simulink model "CRDI_Integrated_Model0707"  (R2019a)
settings: configuration reference "cs1" (kept outside this file)
PreLoadFcn:
  | Configaration_Setting
undefined symbols (not defined in the file or in its folder): AreaOfOrifice_Constant, CcConstant_0, CcConstant_1, Constant_0, Constant_1, Constant_One, Divide_by_100, Error_code_101, Error_code_102, FilterConstant_0, FilterConstant_1, FilterConstant_100, FilterConstant_5, FilterConstant_50, Final_Crank_Angle, Fuel_Discharge, HPPConstant1, HPPConstant2, LPPConstant_0, LPPConstant_1, LPPConstant_10, LPPConstant_3, Main_TgrAng_Inj1, Main_TgrAng_Inj2, Main_TgrAng_Inj3, Main_TgrAng_Inj4, MeterToLiter_Conversion, Orifice_Diameter, Percentage, Pi_value, Post_TgrAng_Inj1, Post_TgrAng_Inj2, Post_TgrAng_Inj3, Post_TgrAng_Inj4, Pre_TgrAng_Inj1, Pre_TgrAng_Inj2, Pre_TgrAng_Inj3, Pre_TgrAng_Inj4, Re_Rounding_Constant, Required_PulseConstant1, Required_PulseConstant2, Required_PulseConstant3, Required_PulseConstant4, resistance_constant, Rounding_Constant_100, Scalling_Factor, Unit_Angle_Compare, Velocity_MulFactor1, Velocity_MulFactor2, Velocity_MulFactor3, Zero_Pulse
libraries: simulink x4
(part 2 of 2)

== system CRDI_Integrated_Model0707/CRDI/Injector_Model/injector1/mainInj1 ==
  Angle : Inport  OutDataTypeStr=single
  Total_On_Time_of_Injector : Inport  Port=2  OutDataTypeStr=single
  Time_For_1_Degree : Inport  Port=3  OutDataTypeStr=single
  Add : Sum  AccumDataTypeStr=single
      settings: AttributesFormatString=AccumDataTypeStr=%<AccumDataTypeStr>
  Constant : Constant  Value=Constant_0
  Constant1 : Constant  Value=Constant_1
  Constant4 : Constant  Value=Main_TgrAng_Inj1
  Constant6 : Constant  Value=Constant_0
  Divide : Product  Inputs=*/  OutDataTypeStr=single
  Logical Operator : Logic  Inputs=3  AllPortsSameDT=off  OutDataTypeStr=boolean
  Relational Operator : RelationalOperator  OutDataTypeStr=boolean  RndMeth=Simplest
  Relational Operator1 : RelationalOperator  Operator=<=  OutDataTypeStr=boolean  RndMeth=Simplest
  Relational Operator2 : RelationalOperator  Operator=>  OutDataTypeStr=boolean  RndMeth=Simplest
  Relational Operator3 : RelationalOperator  Operator=>  OutDataTypeStr=boolean  RndMeth=Simplest
  Switch : Switch  Criteria=u2 ~= 0
  OnPulse_Main : Outport
  wires:
  Switch/1 -> Divide/2  "Time_Of_1_Degree"
  Constant1/1 -> Switch/3  "constant"
  Time_For_1_Degree/1 -> Switch/1, Relational Operator3/1
  [onTinj1] -> Relational Operator2/1
  Total_On_Time_of_Injector/1 -> [onTinj1], Divide/1
  Constant4/1 -> [TrigerAngle], Add/1  "TrigerAngle"
  [TrigerAngle] -> Relational Operator/2
  Relational Operator2/1 -> Logical Operator/3  "Speed_Zero_Or_Not"
  Constant/1 -> Relational Operator2/2  "constant"
  Logical Operator/1 -> OnPulse_Main/1  "OnPulse_Main"
  Divide/1 -> Add/2  "Time_For_On_Pulse"
  Angle/1 -> Relational Operator/1, Relational Operator1/1
  Add/1 -> Relational Operator1/2  "Total_On_Degree"
  Relational Operator/1 -> Logical Operator/1  "Firing_Angle_start"
  Relational Operator1/1 -> Logical Operator/2  "Firing_Angle_Off"
  Relational Operator3/1 -> Switch/2  "Non_Zero_Num"
  Constant6/1 -> Relational Operator3/2  "constant"

== system CRDI_Integrated_Model0707/CRDI/Injector_Model/injector1/postInj1 ==
  Angle : Inport  OutDataTypeStr=single
  Total_On_Time_of_Injector : Inport  Port=2  OutDataTypeStr=single
  Time_for_1_Degree : Inport  Port=3  OutDataTypeStr=single
  Add : Sum  AccumDataTypeStr=single
      settings: AttributesFormatString=AccumDataTypeStr=%<AccumDataTypeStr>
  Constant : Constant  Value=Constant_0
  Constant1 : Constant  Value=Constant_1
  Constant5 : Constant  Value=Post_TgrAng_Inj1
  Constant6 : Constant  Value=Constant_0
  Divide : Product  Inputs=*/  OutDataTypeStr=single
  Logical Operator : Logic  Inputs=3  AllPortsSameDT=off  OutDataTypeStr=boolean
  Relational Operator : RelationalOperator  OutDataTypeStr=boolean  RndMeth=Simplest
  Relational Operator1 : RelationalOperator  Operator=<=  OutDataTypeStr=boolean  RndMeth=Simplest
  Relational Operator2 : RelationalOperator  Operator=>  OutDataTypeStr=boolean  RndMeth=Simplest
  Relational Operator3 : RelationalOperator  Operator=>  OutDataTypeStr=boolean  RndMeth=Simplest
  Switch : Switch  Criteria=u2 ~= 0
  OnPulse_Post : Outport
  wires:
  Time_for_1_Degree/1 -> Relational Operator3/1, Switch/1
  Constant1/1 -> Switch/3  "constant"
  Switch/1 -> Divide/2  "Time_Of_1_Degree"
  Constant5/1 -> Add/1, [TrigerAngle]  "TrigerAngle"
  [TrigerAngle] -> Relational Operator/2
  [onTinj1] -> Relational Operator2/1
  Total_On_Time_of_Injector/1 -> [onTinj1], Divide/1
  Relational Operator2/1 -> Logical Operator/3  "Speed_Zero_Or_Not"
  Constant/1 -> Relational Operator2/2  "constant"
  Logical Operator/1 -> OnPulse_Post/1  "OnPulse_Post"
  Relational Operator1/1 -> Logical Operator/2  "Firing_Angle_Off"
  Relational Operator/1 -> Logical Operator/1  "Firing_Angle_start"
  Add/1 -> Relational Operator1/2  "Total_On_Degree"
  Angle/1 -> Relational Operator/1, Relational Operator1/1
  Divide/1 -> Add/2  "Time_For_On_Pulse"
  Relational Operator3/1 -> Switch/2  "Non_Zero_Num"
  Constant6/1 -> Relational Operator3/2  "constant"

== system CRDI_Integrated_Model0707/CRDI/Injector_Model/injector2/PreInj1 ==
  Angle : Inport  OutDataTypeStr=single
  Total_On_Time_of_Injector : Inport  Port=2  OutDataTypeStr=single
  Time_For_1_Degree : Inport  Port=3  OutDataTypeStr=single
  Add : Sum  AccumDataTypeStr=single
      settings: AttributesFormatString=AccumDataTypeStr=%<AccumDataTypeStr>
  Constant : Constant  Value=Constant_0
  Constant1 : Constant  Value=Constant_1
  Constant2 : Constant  Value=Pre_TgrAng_Inj3  OutDataTypeStr=single
  Constant6 : Constant  Value=Constant_0
  Divide : Product  Inputs=*/  OutDataTypeStr=single
  Logical Operator : Logic  Inputs=3  AllPortsSameDT=off  OutDataTypeStr=boolean
  Relational Operator : RelationalOperator  OutDataTypeStr=boolean  RndMeth=Simplest
  Relational Operator1 : RelationalOperator  Operator=<=  OutDataTypeStr=boolean  RndMeth=Simplest
  Relational Operator2 : RelationalOperator  Operator=>  OutDataTypeStr=boolean  RndMeth=Simplest
  Relational Operator3 : RelationalOperator  Operator=>  OutDataTypeStr=boolean  RndMeth=Simplest
  Switch : Switch  Criteria=u2 ~= 0
  OnPulse_Pre : Outport
  wires:
  Constant1/1 -> Switch/3  "constant"
  Switch/1 -> Divide/2  "Time_Of_1_Degree"
  Constant2/1 -> [TrigerAngle], Add/1  "TrigerAngle"
  [TrigerAngle] -> Relational Operator/2
  [onTinj] -> Relational Operator2/1
  Total_On_Time_of_Injector/1 -> [onTinj], Divide/1
  Constant/1 -> Relational Operator2/2  "constant"
  Relational Operator2/1 -> Logical Operator/3  "Speed_Zero_Or_Not"
  Logical Operator/1 -> OnPulse_Pre/1  "OnPulse_Pre"
  Relational Operator1/1 -> Logical Operator/2  "Firing_Angle_Off"
  Relational Operator/1 -> Logical Operator/1  "Firing_Angle_start"
  Add/1 -> Relational Operator1/2  "Total_On_Degree"
  Angle/1 -> Relational Operator1/1, Relational Operator/1
  Divide/1 -> Add/2  "Time_For_On_Pulse"
  Relational Operator3/1 -> Switch/2  "Non_Zero_Num"
  Constant6/1 -> Relational Operator3/2  "constant"
  Time_For_1_Degree/1 -> Switch/1, Relational Operator3/1

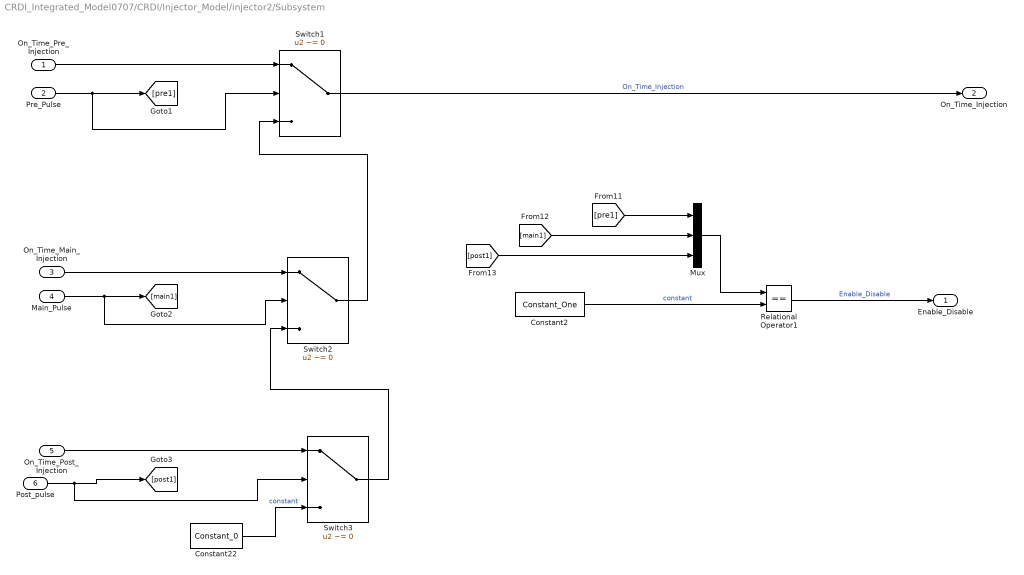
== system CRDI_Integrated_Model0707/CRDI/Injector_Model/injector2/Subsystem ==
  On_Time_Pre_Injection : Inport
  Pre_Pulse : Inport  Port=2
  On_Time_Main_Injection : Inport  Port=3
  Main_Pulse : Inport  Port=4
  On_Time_Post_Injection : Inport  Port=5
  Post_pulse : Inport  Port=6
  Constant2 : Constant  Value=Constant_One  OutDataTypeStr=single
  Constant22 : Constant  Value=Constant_0  OutDataTypeStr=single
  Mux : Mux  Inputs=3
  Relational Operator1 : RelationalOperator  Operator===  OutDataTypeStr=boolean  RndMeth=Simplest
  Switch1 : Switch  Criteria=u2 ~= 0
  Switch2 : Switch  Criteria=u2 ~= 0
  Switch3 : Switch  Criteria=u2 ~= 0
  Enable_Disable : Outport
  On_Time_Injection : Outport  Port=2
  wires:
  Post_pulse/1 -> [post1], Switch3/2
  On_Time_Post_Injection/1 -> Switch3/1
  Main_Pulse/1 -> [main1], Switch2/2
  On_Time_Main_Injection/1 -> Switch2/1
  Pre_Pulse/1 -> [pre1], Switch1/2
  On_Time_Pre_Injection/1 -> Switch1/1
  Switch1/1 -> On_Time_Injection/1  "On_Time_Injection"
  Relational Operator1/1 -> Enable_Disable/1  "Enable_Disable"
  Constant22/1 -> Switch3/3  "constant"
  [main1] -> Mux/2
  Switch3/1 -> Switch2/3
  Switch2/1 -> Switch1/3
  Mux/1 -> Relational Operator1/1
  [pre1] -> Mux/1
  [post1] -> Mux/3
  Constant2/1 -> Relational Operator1/2  "constant"

== system CRDI_Integrated_Model0707/CRDI/Injector_Model/injector2/Subsystem7 ==
  On_Time : Inport
  Enable : EnablePort  StatesWhenEnabling=reset  PropagateVarSize=During execution
  Add : Sum  AccumDataTypeStr=single
      settings: AttributesFormatString=AccumDataTypeStr=%<AccumDataTypeStr>
  Constant : Constant  Value=Re_Rounding_Constant  OutDataTypeStr=single
  Relational Operator : RelationalOperator  Operator=<=  OutDataTypeStr=boolean  RndMeth=Simplest
  Subsystem : Subsystem  Commented=on
  Unit Delay : UnitDelay  SampleTime=-1  HasFrameUpgradeWarning=on
  Final_Inj_Pulse : Outport  OutDataTypeStr=boolean
  wires:
  Relational Operator/1 -> Final_Inj_Pulse/1  "Final_Inj_Pulse"
  Unit Delay/1 -> Add/1
  Constant/1 -> Add/2  "constant"
  Add/1 -> Relational Operator/1, Unit Delay/1
  On_Time/1 -> Relational Operator/2

== system CRDI_Integrated_Model0707/CRDI/Injector_Model/injector2/mainInj1 ==
  Angle : Inport  OutDataTypeStr=single
  Total_On_Time_of_Injector : Inport  Port=2  OutDataTypeStr=single
  Time_For_1_Degree : Inport  Port=3  OutDataTypeStr=single
  Add : Sum  AccumDataTypeStr=single
      settings: AttributesFormatString=AccumDataTypeStr=%<AccumDataTypeStr>
  Constant : Constant  Value=Constant_0
  Constant1 : Constant  Value=Constant_1
  Constant4 : Constant  Value=Main_TgrAng_Inj3
  Constant6 : Constant  Value=Constant_0
  Divide : Product  Inputs=*/  OutDataTypeStr=single
  Logical Operator : Logic  Inputs=3  AllPortsSameDT=off  OutDataTypeStr=boolean
  Relational Operator : RelationalOperator  OutDataTypeStr=boolean  RndMeth=Simplest
  Relational Operator1 : RelationalOperator  Operator=<=  OutDataTypeStr=boolean  RndMeth=Simplest
  Relational Operator2 : RelationalOperator  Operator=>  OutDataTypeStr=boolean  RndMeth=Simplest
  Relational Operator3 : RelationalOperator  Operator=>  OutDataTypeStr=boolean  RndMeth=Simplest
  Switch : Switch  Criteria=u2 ~= 0
  OnPulse_Main : Outport
  wires:
  Switch/1 -> Divide/2  "Time_Of_1_Degree"
  Constant1/1 -> Switch/3  "constant"
  [onTinj1] -> Relational Operator2/1
  Total_On_Time_of_Injector/1 -> [onTinj1], Divide/1
  Constant4/1 -> [TrigerAngle], Add/1  "TrigerAngle"
  [TrigerAngle] -> Relational Operator/2
  Relational Operator2/1 -> Logical Operator/3  "Speed_Zero_Or_Not"
  Constant/1 -> Relational Operator2/2  "constant"
  Logical Operator/1 -> OnPulse_Main/1  "OnPulse_Main"
  Divide/1 -> Add/2  "Time_For_On_Pulse"
  Angle/1 -> Relational Operator/1, Relational Operator1/1
  Add/1 -> Relational Operator1/2  "Total_On_Degree"
  Relational Operator/1 -> Logical Operator/1  "Firing_Angle_start"
  Relational Operator1/1 -> Logical Operator/2  "Firing_Angle_Off"
  Relational Operator3/1 -> Switch/2  "Non_Zero_Num"
  Constant6/1 -> Relational Operator3/2  "constant"
  Time_For_1_Degree/1 -> Switch/1, Relational Operator3/1

== system CRDI_Integrated_Model0707/CRDI/Injector_Model/injector2/postInj1 ==
  Angle : Inport  OutDataTypeStr=single
  Total_On_Time_of_Injector : Inport  Port=2  OutDataTypeStr=single
  Time_for_1_Degree : Inport  Port=3  OutDataTypeStr=single
  Add : Sum  AccumDataTypeStr=single
      settings: AttributesFormatString=AccumDataTypeStr=%<AccumDataTypeStr>
  Constant : Constant  Value=Constant_0
  Constant1 : Constant  Value=Constant_1
  Constant5 : Constant  Value=Post_TgrAng_Inj3
  Constant6 : Constant  Value=Constant_0
  Divide : Product  Inputs=*/  OutDataTypeStr=single
  Logical Operator : Logic  Inputs=3  AllPortsSameDT=off  OutDataTypeStr=boolean
  Relational Operator : RelationalOperator  OutDataTypeStr=boolean  RndMeth=Simplest
  Relational Operator1 : RelationalOperator  Operator=<=  OutDataTypeStr=boolean  RndMeth=Simplest
  Relational Operator2 : RelationalOperator  Operator=>  OutDataTypeStr=boolean  RndMeth=Simplest
  Relational Operator3 : RelationalOperator  Operator=>  OutDataTypeStr=boolean  RndMeth=Simplest
  Switch : Switch  Criteria=u2 ~= 0
  OnPulse_Post : Outport
  wires:
  Constant1/1 -> Switch/3  "constant"
  Switch/1 -> Divide/2  "Time_Of_1_Degree"
  Constant5/1 -> Add/1, [TrigerAngle]  "TrigerAngle"
  [TrigerAngle] -> Relational Operator/2
  [onTinj1] -> Relational Operator2/1
  Total_On_Time_of_Injector/1 -> [onTinj1], Divide/1
  Relational Operator2/1 -> Logical Operator/3  "Speed_Zero_Or_Not"
  Constant/1 -> Relational Operator2/2  "constant"
  Logical Operator/1 -> OnPulse_Post/1  "OnPulse_Post"
  Relational Operator1/1 -> Logical Operator/2  "Firing_Angle_Off"
  Relational Operator/1 -> Logical Operator/1  "Firing_Angle_start"
  Add/1 -> Relational Operator1/2  "Total_On_Degree"
  Angle/1 -> Relational Operator/1, Relational Operator1/1
  Divide/1 -> Add/2  "Time_For_On_Pulse"
  Relational Operator3/1 -> Switch/2  "Non_Zero_Num"
  Constant6/1 -> Relational Operator3/2  "constant"
  Time_for_1_Degree/1 -> Switch/1, Relational Operator3/1

== system CRDI_Integrated_Model0707/CRDI/Injector_Model/injector3/PreInj1 ==
  Angle : Inport  OutDataTypeStr=single
  Total_On_Time_of_Injector : Inport  Port=2  OutDataTypeStr=single
  Time_For_1_Degree : Inport  Port=3  OutDataTypeStr=single
  Add : Sum  AccumDataTypeStr=single
      settings: AttributesFormatString=AccumDataTypeStr=%<AccumDataTypeStr>
  Constant : Constant  Value=Constant_0
  Constant1 : Constant  Value=Constant_1
  Constant6 : Constant  Value=Constant_0
  Constant9 : Constant  Value=Pre_TgrAng_Inj2  OutDataTypeStr=single
  Divide : Product  Inputs=*/  OutDataTypeStr=single
  Logical Operator : Logic  Inputs=3  AllPortsSameDT=off  OutDataTypeStr=boolean
  Relational Operator : RelationalOperator  OutDataTypeStr=boolean  RndMeth=Simplest
  Relational Operator1 : RelationalOperator  Operator=<=  OutDataTypeStr=boolean  RndMeth=Simplest
  Relational Operator2 : RelationalOperator  Operator=>  OutDataTypeStr=boolean  RndMeth=Simplest
  Relational Operator3 : RelationalOperator  Operator=>  OutDataTypeStr=boolean  RndMeth=Simplest
  Switch : Switch  Criteria=u2 ~= 0
  OnPulse_Pre : Outport
  wires:
  Time_For_1_Degree/1 -> Switch/1, Relational Operator3/1
  Constant1/1 -> Switch/3  "constant"
  Switch/1 -> Divide/2  "Time_Of_1_Degree"
  Constant9/1 -> [TrigerAngle], Add/1  "TrigerAngle"
  [TrigerAngle] -> Relational Operator/2
  [onTinj] -> Relational Operator2/1
  Total_On_Time_of_Injector/1 -> [onTinj], Divide/1
  Constant/1 -> Relational Operator2/2  "constant"
  Relational Operator2/1 -> Logical Operator/3  "Speed_Zero_Or_Not"
  Logical Operator/1 -> OnPulse_Pre/1  "OnPulse_Pre"
  Relational Operator1/1 -> Logical Operator/2  "Firing_Angle_Off"
  Relational Operator/1 -> Logical Operator/1  "Firing_Angle_start"
  Add/1 -> Relational Operator1/2  "Total_On_Degree"
  Angle/1 -> Relational Operator1/1, Relational Operator/1
  Divide/1 -> Add/2  "Time_For_On_Pulse"
  Relational Operator3/1 -> Switch/2  "Non_Zero_Num"
  Constant6/1 -> Relational Operator3/2  "constant"

== system CRDI_Integrated_Model0707/CRDI/Injector_Model/injector3/Subsystem ==
  On_Time_Pre_Injection : Inport
  Pre_Pulse : Inport  Port=2
  On_Time_Main_Injection : Inport  Port=3
  Main_Pulse : Inport  Port=4
  On_Time_Post_Injection : Inport  Port=5
  Post_pulse : Inport  Port=6
  Constant2 : Constant  Value=Constant_One  OutDataTypeStr=single
  Constant22 : Constant  Value=Constant_0  OutDataTypeStr=single
  Mux : Mux  Inputs=3
  Relational Operator1 : RelationalOperator  Operator===  OutDataTypeStr=boolean  RndMeth=Simplest
  Switch1 : Switch  Criteria=u2 ~= 0
  Switch2 : Switch  Criteria=u2 ~= 0
  Switch3 : Switch  Criteria=u2 ~= 0
  Enable_Disable : Outport
  On_Time_Injection : Outport  Port=2
  wires:
  Post_pulse/1 -> [post1], Switch3/2
  On_Time_Post_Injection/1 -> Switch3/1
  Main_Pulse/1 -> [main1], Switch2/2
  On_Time_Main_Injection/1 -> Switch2/1
  Pre_Pulse/1 -> [pre1], Switch1/2
  On_Time_Pre_Injection/1 -> Switch1/1
  Switch1/1 -> On_Time_Injection/1  "On_Time_Injection"
  Relational Operator1/1 -> Enable_Disable/1  "Enable_Disable"
  Constant22/1 -> Switch3/3  "constant"
  [main1] -> Mux/2
  Constant2/1 -> Relational Operator1/2  "constant"
  Switch3/1 -> Switch2/3
  Switch2/1 -> Switch1/3
  Mux/1 -> Relational Operator1/1
  [pre1] -> Mux/1
  [post1] -> Mux/3

== system CRDI_Integrated_Model0707/CRDI/Injector_Model/injector3/Subsystem7 ==
  On_Time : Inport
  Enable : EnablePort  StatesWhenEnabling=reset  PropagateVarSize=During execution
  Add : Sum  AccumDataTypeStr=single
      settings: AttributesFormatString=AccumDataTypeStr=%<AccumDataTypeStr>
  Constant : Constant  Value=Re_Rounding_Constant  OutDataTypeStr=single
  Relational Operator : RelationalOperator  Operator=<=  OutDataTypeStr=boolean  RndMeth=Simplest
  Subsystem : Subsystem  Commented=on
  Unit Delay : UnitDelay  SampleTime=-1  HasFrameUpgradeWarning=on
  Final_Inj_Pulse : Outport  OutDataTypeStr=boolean
  wires:
  Relational Operator/1 -> Final_Inj_Pulse/1  "Final_Inj_Pulse"
  Unit Delay/1 -> Add/1
  Constant/1 -> Add/2  "constant"
  Add/1 -> Relational Operator/1, Unit Delay/1
  On_Time/1 -> Relational Operator/2

== system CRDI_Integrated_Model0707/CRDI/Injector_Model/injector3/mainInj1 ==
  Angle : Inport  OutDataTypeStr=single
  Total_On_Time_of_Injector : Inport  Port=2  OutDataTypeStr=single
  Time_For_1_Degree : Inport  Port=3  OutDataTypeStr=single
  Add : Sum  AccumDataTypeStr=single
      settings: AttributesFormatString=AccumDataTypeStr=%<AccumDataTypeStr>
  Constant : Constant  Value=Constant_0
  Constant1 : Constant  Value=Constant_1
  Constant11 : Constant  Value=Main_TgrAng_Inj2  OutDataTypeStr=single
  Constant6 : Constant  Value=Constant_0
  Divide : Product  Inputs=*/  OutDataTypeStr=single
  Logical Operator : Logic  Inputs=3  AllPortsSameDT=off  OutDataTypeStr=boolean
  Relational Operator : RelationalOperator  OutDataTypeStr=boolean  RndMeth=Simplest
  Relational Operator1 : RelationalOperator  Operator=<=  OutDataTypeStr=boolean  RndMeth=Simplest
  Relational Operator2 : RelationalOperator  Operator=>  OutDataTypeStr=boolean  RndMeth=Simplest
  Relational Operator3 : RelationalOperator  Operator=>  OutDataTypeStr=boolean  RndMeth=Simplest
  Switch : Switch  Criteria=u2 ~= 0
  OnPulse_Main : Outport
  wires:
  Switch/1 -> Divide/2  "Time_Of_1_Degree"
  Constant1/1 -> Switch/3  "constant"
  Time_For_1_Degree/1 -> Relational Operator3/1, Switch/1
  [onTinj1] -> Relational Operator2/1
  Total_On_Time_of_Injector/1 -> [onTinj1], Divide/1
  Constant11/1 -> [TrigerAngle], Add/1  "TrigerAngle"
  [TrigerAngle] -> Relational Operator/2
  Relational Operator2/1 -> Logical Operator/3  "Speed_Zero_Or_Not"
  Constant/1 -> Relational Operator2/2  "constant"
  Logical Operator/1 -> OnPulse_Main/1  "OnPulse_Main"
  Divide/1 -> Add/2  "Time_For_On_Pulse"
  Angle/1 -> Relational Operator/1, Relational Operator1/1
  Add/1 -> Relational Operator1/2  "Total_On_Degree"
  Relational Operator/1 -> Logical Operator/1  "Firing_Angle_start"
  Relational Operator1/1 -> Logical Operator/2  "Firing_Angle_Off"
  Relational Operator3/1 -> Switch/2  "Non_Zero_Num"
  Constant6/1 -> Relational Operator3/2  "constant"

== system CRDI_Integrated_Model0707/CRDI/Injector_Model/injector3/postInj1 ==
  Angle : Inport  OutDataTypeStr=single
  Total_On_Time_of_Injector : Inport  Port=2  OutDataTypeStr=single
  Time_for_1_Degree : Inport  Port=3  OutDataTypeStr=single
  Add : Sum  AccumDataTypeStr=single
      settings: AttributesFormatString=AccumDataTypeStr=%<AccumDataTypeStr>
  Constant : Constant  Value=Constant_0
  Constant1 : Constant  Value=Constant_1
  Constant12 : Constant  Value=Post_TgrAng_Inj2
  Constant6 : Constant  Value=Constant_0
  Divide : Product  Inputs=*/  OutDataTypeStr=single
  Logical Operator : Logic  Inputs=3  AllPortsSameDT=off  OutDataTypeStr=boolean
  Relational Operator : RelationalOperator  OutDataTypeStr=boolean  RndMeth=Simplest
  Relational Operator1 : RelationalOperator  Operator=<=  OutDataTypeStr=boolean  RndMeth=Simplest
  Relational Operator2 : RelationalOperator  Operator=>  OutDataTypeStr=boolean  RndMeth=Simplest
  Relational Operator3 : RelationalOperator  Operator=>  OutDataTypeStr=boolean  RndMeth=Simplest
  Switch : Switch  Criteria=u2 ~= 0
  OnPulse_Post : Outport
  wires:
  Time_for_1_Degree/1 -> Relational Operator3/1, Switch/1
  Constant1/1 -> Switch/3  "constant"
  Switch/1 -> Divide/2  "Time_Of_1_Degree"
  Constant12/1 -> Add/1, [TrigerAngle]  "TrigerAngle"
  [TrigerAngle] -> Relational Operator/2
  [onTinj1] -> Relational Operator2/1
  Total_On_Time_of_Injector/1 -> [onTinj1], Divide/1
  Relational Operator2/1 -> Logical Operator/3  "Speed_Zero_Or_Not"
  Constant/1 -> Relational Operator2/2  "constant"
  Logical Operator/1 -> OnPulse_Post/1  "OnPulse_Post"
  Relational Operator1/1 -> Logical Operator/2  "Firing_Angle_Off"
  Relational Operator/1 -> Logical Operator/1  "Firing_Angle_start"
  Add/1 -> Relational Operator1/2  "Total_On_Degree"
  Angle/1 -> Relational Operator/1, Relational Operator1/1
  Divide/1 -> Add/2  "Time_For_On_Pulse"
  Relational Operator3/1 -> Switch/2  "Non_Zero_Num"
  Constant6/1 -> Relational Operator3/2  "constant"

== system CRDI_Integrated_Model0707/CRDI/Injector_Model/injector4/MainInj4 ==
  angle : Inport  OutDataTypeStr=single
  total_on_time_of_injector : Inport  Port=2  OutDataTypeStr=single
  time_for_1_degree : Inport  Port=3  OutDataTypeStr=single
  speed : Inport  Port=4  OutDataTypeStr=single
  Add : Sum  AccumDataTypeStr=single
      settings: AttributesFormatString=AccumDataTypeStr=%<AccumDataTypeStr>
  Constant : Constant  OutDataTypeStr=single
  Constant1 : Constant  Value=Constant_0
  Constant2 : Constant  Value=Constant_1
  Constant23 : Constant  Value=Main_TgrAng_Inj4
  Constant6 : Constant  Value=Constant_0
  Display : Display
  Display1 : Display
  Display2 : Display
  Divide : Product  Inputs=*/  OutDataTypeStr=single
  Relational Operator : RelationalOperator  Operator===  OutDataTypeStr=boolean  RndMeth=Simplest
  Relational Operator1 : RelationalOperator  Operator=<=  OutDataTypeStr=boolean  RndMeth=Simplest
  Relational Operator2 : RelationalOperator  Operator=>  OutDataTypeStr=boolean  RndMeth=Simplest
  Relational Operator3 : RelationalOperator  Operator=>  OutDataTypeStr=boolean  RndMeth=Simplest
  Switch : Switch  Criteria=u2 ~= 0
  OnPulse_Post : Outport  OutDataTypeStr=boolean
  wires:
  total_on_time_of_injector/1 -> Divide/1
  Divide/1 -> Add/2  "Time_For_On_Pulse"
  angle/1 -> Relational Operator1/1, Relational Operator/1
  Constant23/1 -> Relational Operator/2  "TrigerAngle"
  Add/1 -> Relational Operator1/2  "Total_On_Degree"
  Constant/1 -> Add/1  "constant"
  Constant1/1 -> Relational Operator2/2  "constant"
  speed/1 -> Relational Operator2/1
  Relational Operator/1 -> Display/1  "Equal"
  Relational Operator2/1 -> Display2/1  "Speed_Zero"
  Relational Operator1/1 -> OnPulse_Post/1, Display1/1  "OnPulse_Post"
  Switch/1 -> Divide/2
  Constant2/1 -> Switch/3  "constant"
  time_for_1_degree/1 -> Relational Operator3/1, Switch/1
  Relational Operator3/1 -> Switch/2  "Non_Zero_Num"
  Constant6/1 -> Relational Operator3/2  "constant"

== system CRDI_Integrated_Model0707/CRDI/Injector_Model/injector4/On_Time_Injector ==
  On_Time_Pre_Inj : Inport
  Pre_Pulse : Inport  Port=2
  On_Time_Main_Inj : Inport  Port=3
  Main_Pulse : Inport  Port=4
  On_Time_Post_Inj : Inport  Port=5
  Post_pulse : Inport  Port=6
  Constant22 : Constant  Value=Constant_0  OutDataTypeStr=single
  Constant3 : Constant  Value=Constant_One  OutDataTypeStr=single
  Mux : Mux  Inputs=3
  Relational Operator1 : RelationalOperator  Operator===  OutDataTypeStr=boolean  RndMeth=Simplest
  Switch1 : Switch  Criteria=u2 ~= 0
  Switch2 : Switch  Criteria=u2 ~= 0
  Switch3 : Switch  Criteria=u2 ~= 0
  Enable_Disable : Outport
  On_Time_injector : Outport  Port=2
  wires:
  [pre1] -> Mux/1
  [main1] -> Mux/2
  Switch3/1 -> Switch2/3  "OTPI"
  Post_pulse/1 -> Switch3/2, [post1]
  Switch1/1 -> On_Time_injector/1  "On_Time_injector"
  [post1] -> Mux/3
  Relational Operator1/1 -> Enable_Disable/1  "Enable_Disable"
  Main_Pulse/1 -> Switch2/2, [main1]
  On_Time_Pre_Inj/1 -> Switch1/1
  Pre_Pulse/1 -> Switch1/2, [pre1]
  Constant22/1 -> Switch3/3  "constant"
  Constant3/1 -> Relational Operator1/2  "constant"
  Switch2/1 -> Switch1/3  "OTMI"
  Mux/1 -> Relational Operator1/1  "Bus"
  On_Time_Main_Inj/1 -> Switch2/1
  On_Time_Post_Inj/1 -> Switch3/1

== system CRDI_Integrated_Model0707/CRDI/Injector_Model/injector4/PostInj4 ==
  angle : Inport  OutDataTypeStr=single
  total_on_time_of_injector : Inport  Port=2  OutDataTypeStr=single
  time_for_1_degree : Inport  Port=3  OutDataTypeStr=single
  Add : Sum  AccumDataTypeStr=single
      settings: AttributesFormatString=AccumDataTypeStr=%<AccumDataTypeStr>
  Constant : Constant  Value=Constant_0
  Constant1 : Constant  Value=Constant_1
  Constant24 : Constant  Value=Post_TgrAng_Inj4
  Constant6 : Constant  Value=Constant_0
  Divide : Product  Inputs=*/  OutDataTypeStr=single
  Logical Operator : Logic  Inputs=3  AllPortsSameDT=off  OutDataTypeStr=boolean
  Relational Operator : RelationalOperator  OutDataTypeStr=boolean  RndMeth=Simplest
  Relational Operator1 : RelationalOperator  Operator=<=  OutDataTypeStr=boolean  RndMeth=Simplest
  Relational Operator2 : RelationalOperator  Operator=>  OutDataTypeStr=boolean  RndMeth=Simplest
  Relational Operator3 : RelationalOperator  Operator=>  OutDataTypeStr=boolean  RndMeth=Simplest
  Switch : Switch  Criteria=u2 ~= 0
  OnPulse_Post : Outport  OutDataTypeStr=boolean
  wires:
  Logical Operator/1 -> OnPulse_Post/1  "OnPulse_Post"
  Relational Operator1/1 -> Logical Operator/2  "Rel_Op"
  Relational Operator/1 -> Logical Operator/1  "Rel_Op"
  Add/1 -> Relational Operator1/2  "Total_On_Degree"
  angle/1 -> Relational Operator1/1, Relational Operator/1
  Divide/1 -> Add/2  "Time_For_On_Pulse"
  Constant/1 -> Relational Operator2/2  "constant"
  Relational Operator2/1 -> Logical Operator/3  "Rel_Op"
  [TrigerAngle] -> Relational Operator/2
  Constant24/1 -> Add/1, [TrigerAngle]  "TrigerAngle"
  total_on_time_of_injector/1 -> Divide/1, [onTinj1]
  [onTinj1] -> Relational Operator2/1
  Switch/1 -> Divide/2  "T1D"
  Constant1/1 -> Switch/3  "constant"
  time_for_1_degree/1 -> Relational Operator3/1, Switch/1
  Relational Operator3/1 -> Switch/2  "Non_Zero_Num"
  Constant6/1 -> Relational Operator3/2  "constant"

== system CRDI_Integrated_Model0707/CRDI/Injector_Model/injector4/PreInj4 ==
  angle : Inport  OutDataTypeStr=single
  total_on_time_of_injector : Inport  Port=2  OutDataTypeStr=single
  time_for_1_degree : Inport  Port=3  OutDataTypeStr=single
  Add : Sum  AccumDataTypeStr=single
      settings: AttributesFormatString=AccumDataTypeStr=%<AccumDataTypeStr>
  Constant : Constant  Value=Constant_0
  Constant1 : Constant  Value=Constant_1
  Constant28 : Constant  Value=Pre_TgrAng_Inj4
  Constant6 : Constant  Value=Constant_0
  Divide : Product  Inputs=*/  OutDataTypeStr=single
  Logical Operator : Logic  Inputs=3  AllPortsSameDT=off  OutDataTypeStr=boolean
  Relational Operator : RelationalOperator  OutDataTypeStr=boolean  RndMeth=Simplest
  Relational Operator1 : RelationalOperator  Operator=<=  OutDataTypeStr=boolean  RndMeth=Simplest
  Relational Operator2 : RelationalOperator  Operator=>  OutDataTypeStr=boolean  RndMeth=Simplest
  Relational Operator3 : RelationalOperator  Operator=>  OutDataTypeStr=boolean  RndMeth=Simplest
  Switch : Switch  Criteria=u2 ~= 0
  OnPulse_Pre : Outport  OutDataTypeStr=boolean
  wires:
  Logical Operator/1 -> OnPulse_Pre/1  "OnPulse_Pre"
  Relational Operator1/1 -> Logical Operator/2  "Firing_Angle_Stop"
  Relational Operator/1 -> Logical Operator/1  "fFiring_Angle_Start"
  Add/1 -> Relational Operator1/2  "Total_On_Degree"
  angle/1 -> Relational Operator/1, Relational Operator1/1
  Divide/1 -> Add/2  "Time_For_On_Pulse"
  Constant/1 -> Relational Operator2/2  "constant"
  Relational Operator2/1 -> Logical Operator/3  "Speed_Zero"
  [TrigerAngle] -> Relational Operator/2
  Constant28/1 -> Add/1, [TrigerAngle]  "TrigerAngle"
  total_on_time_of_injector/1 -> Divide/1, [onTinj1]
  [onTinj1] -> Relational Operator2/1
  Switch/1 -> Divide/2
  Constant1/1 -> Switch/3  "constant"
  time_for_1_degree/1 -> Relational Operator3/1, Switch/1
  Relational Operator3/1 -> Switch/2  "Non_Zero_Num"
  Constant6/1 -> Relational Operator3/2  "constant"

== system CRDI_Integrated_Model0707/CRDI/Injector_Model/injector4/Subsystem7 ==
  on_time : Inport  OutDataTypeStr=single
  Enable : EnablePort  StatesWhenEnabling=reset  PropagateVarSize=During execution
  Add : Sum  AccumDataTypeStr=single
      settings: AttributesFormatString=AccumDataTypeStr=%<AccumDataTypeStr>
  Constant : Constant  Value=Re_Rounding_Constant  OutDataTypeStr=single
  Relational Operator : RelationalOperator  Operator=<=  OutDataTypeStr=boolean  RndMeth=Simplest
  Subsystem : Subsystem  Commented=on
  Unit Delay : UnitDelay  SampleTime=-1  HasFrameUpgradeWarning=on
  Inj4pulse : Outport  OutDataTypeStr=boolean
  wires:
  Unit Delay/1 -> Add/1
  Constant/1 -> Add/2  "constant"
  Add/1 -> Relational Operator/1, Unit Delay/1
  Relational Operator/1 -> Inj4pulse/1  "Inj4pulse"
  on_time/1 -> Relational Operator/2

== system CRDI_Integrated_Model0707/CRDI/Injector_Model/injector1/Subsystem7/Subsystem ==
  In1 : Inport
  In2 : Inport  Port=2
  In3 : Inport  Port=3
  Constant1 : Constant  Commented=on  Value=Constant_0  OutDataTypeStr=single
  Constant2 : Constant  Commented=on  Value=Rounding_Constant_100
  Constant3 : Constant  Commented=on  Value=Re_Rounding_Constant
  Product : Product  Commented=on  OutDataTypeStr=single
  Product1 : Product  Commented=on  OutDataTypeStr=single
  Round : Rounding  Commented=on  Operator=round
      settings: AttributesFormatString=Operator=%<Operator>
  Switch1 : Switch  Commented=on  Criteria=u2 ~= 0
  Out1 : Outport
  Out2 : Outport  Port=2
  wires:
  Switch1/1 -> Out2/1
  In2/1 -> Switch1/1
  Product1/1 -> Out1/1
  In1/1 -> Product/1
  Round/1 -> Product1/1
  Product/1 -> Round/1
  Constant1/1 -> Switch1/3
  Constant3/1 -> Product1/2
  Constant2/1 -> Product/2
  In3/1 -> Switch1/2

== system CRDI_Integrated_Model0707/CRDI/Injector_Model/injector2/Subsystem7/Subsystem ==
  In1 : Inport
  In2 : Inport  Port=2
  In3 : Inport  Port=3
  Constant1 : Constant  Commented=on  Value=Constant_0  OutDataTypeStr=single
  Constant2 : Constant  Commented=on  Value=Rounding_Constant_100
  Constant3 : Constant  Commented=on  Value=Re_Rounding_Constant
  Product : Product  Commented=on  OutDataTypeStr=single
  Product1 : Product  Commented=on  OutDataTypeStr=single
  Round : Rounding  Commented=on  Operator=round
      settings: AttributesFormatString=Operator=%<Operator>
  Switch1 : Switch  Commented=on  Criteria=u2 ~= 0
  Out1 : Outport
  Out2 : Outport  Port=2
  wires:
  Switch1/1 -> Out2/1
  In2/1 -> Switch1/1
  Product1/1 -> Out1/1
  In1/1 -> Product/1
  Round/1 -> Product1/1
  Product/1 -> Round/1
  Constant1/1 -> Switch1/3
  Constant3/1 -> Product1/2
  Constant2/1 -> Product/2
  In3/1 -> Switch1/2

== system CRDI_Integrated_Model0707/CRDI/Injector_Model/injector3/Subsystem7/Subsystem ==
  In1 : Inport
  In2 : Inport  Port=2
  In3 : Inport  Port=3
  Constant1 : Constant  Commented=on  Value=Constant_0  OutDataTypeStr=single
  Constant2 : Constant  Commented=on  Value=Rounding_Constant_100
  Constant3 : Constant  Commented=on  Value=Re_Rounding_Constant
  Product : Product  Commented=on  OutDataTypeStr=single
  Product1 : Product  Commented=on  OutDataTypeStr=single
  Round : Rounding  Commented=on  Operator=round
      settings: AttributesFormatString=Operator=%<Operator>
  Switch1 : Switch  Commented=on  Criteria=u2 ~= 0
  Out1 : Outport
  Out2 : Outport  Port=2
  wires:
  Switch1/1 -> Out2/1
  In2/1 -> Switch1/1
  Product1/1 -> Out1/1
  In1/1 -> Product/1
  Round/1 -> Product1/1
  Product/1 -> Round/1
  Constant1/1 -> Switch1/3
  Constant3/1 -> Product1/2
  Constant2/1 -> Product/2
  In3/1 -> Switch1/2

== system CRDI_Integrated_Model0707/CRDI/Injector_Model/injector4/Subsystem7/Subsystem ==
  In1 : Inport
  In2 : Inport  Port=2
  In3 : Inport  Port=3
  Constant1 : Constant  Commented=on  Value=Re_Rounding_Constant  OutDataTypeStr=single
  Constant2 : Constant  Commented=on  Value=Rounding_Constant_100
  Constant3 : Constant  Commented=on  Value=Constant_0  OutDataTypeStr=single
  Product : Product  Commented=on  OutDataTypeStr=single
  Product1 : Product  Commented=on  OutDataTypeStr=single
  Round : Rounding  Commented=on  Operator=round
      settings: AttributesFormatString=Operator=%<Operator>
  Switch1 : Switch  Commented=on  Criteria=u2 ~= 0
  Out1 : Outport
  Out2 : Outport  Port=2
  wires:
  Constant3/1 -> Switch1/3
  Constant2/1 -> Product/2
  Product/1 -> Round/1
  Round/1 -> Product1/1
  Constant1/1 -> Product1/2
  In2/1 -> Switch1/1
  In3/1 -> Switch1/2
  Switch1/1 -> Out2/1
  In1/1 -> Product/1
  Product1/1 -> Out1/1
